simulink model "Opm"  (Simulink 8.4)
settings: Solver=ode45  StartTime=0.0  StopTime=10.0  RelTol=1e-3
undefined symbols (not defined in the file): Opm_stDiagnosisOverride, Opm_stEngControl, Opm_stIOErrorOverride, Opm_tiIOErrorDelay
libraries: simulink x1
settings Model: Creator=YAL9FE  LastModifiedBy=ric9fe
settings DebuggingCC: FcnCallInpInsideContextMsg=EnableAllAsWarning

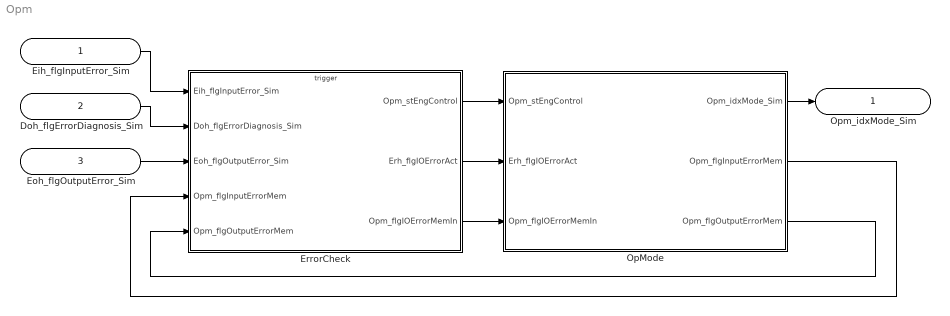
== system Opm ==
  Eih_flgInputError_Sim : Inport
  Doh_flgErrorDiagnosis_Sim : Inport  Port=2
  Eoh_flgOutputError_Sim : Inport  Port=3
  ErrorCheck : Subsystem  mask(Functions){}
      mask help: ErrorCheck
      mask Display:
      | image(imread('OperationMode.jpg'))
      | port_label('input',1,'Eih_flgInputError_Sim')
      | port_label('input',2,'Doh_flgErrorDiagnosis_Sim')
      | port_label('input',3,'Eoh_flgOutputError_Sim')
      | port_label('input',4,'Opm_flgInputErrorMem')
      | port_label('input',5,'Opm_flgOutputErrorMem')
      | port_label('output',1,'Opm_stEngControl')
      | port_label('output',2,'Erh_flgIOErrorAct')
      | port_label('output',3,'Opm_flgIOErrorMemIn')
  OpMode : Subsystem  mask(Functions){}
      mask help: OpMode
      mask Display:
      | image(imread('OperationMode.jpg'))
      | port_label('input',1,'Opm_stEngControl')
      | port_label('input',2,'Erh_flgIOErrorAct')
      | port_label('input',3,'Opm_flgIOErrorMemIn')
      | port_label('output',1,'Opm_idxMode_Sim')
      | port_label('output',2,'Opm_flgInputErrorMem')
      | port_label('output',3,'Opm_flgOutputErrorMem')
  Opm_idxMode_Sim : Outport
  wires:
  Eih_flgInputError_Sim/1 -> ErrorCheck/1(Eih_flgInputError_Sim)
  Doh_flgErrorDiagnosis_Sim/1 -> ErrorCheck/2(Doh_flgErrorDiagnosis_Sim)
  Eoh_flgOutputError_Sim/1 -> ErrorCheck/3(Eoh_flgOutputError_Sim)
  OpMode/1(Opm_idxMode_Sim) -> Opm_idxMode_Sim/1
  ErrorCheck/1(Opm_stEngControl) -> OpMode/1(Opm_stEngControl)
  ErrorCheck/2(Erh_flgIOErrorAct) -> OpMode/2(Erh_flgIOErrorAct)
  ErrorCheck/3(Opm_flgIOErrorMemIn) -> OpMode/3(Opm_flgIOErrorMemIn)
  OpMode/2(Opm_flgInputErrorMem) -> ErrorCheck/4(Opm_flgInputErrorMem)
  OpMode/3(Opm_flgOutputErrorMem) -> ErrorCheck/5(Opm_flgOutputErrorMem)

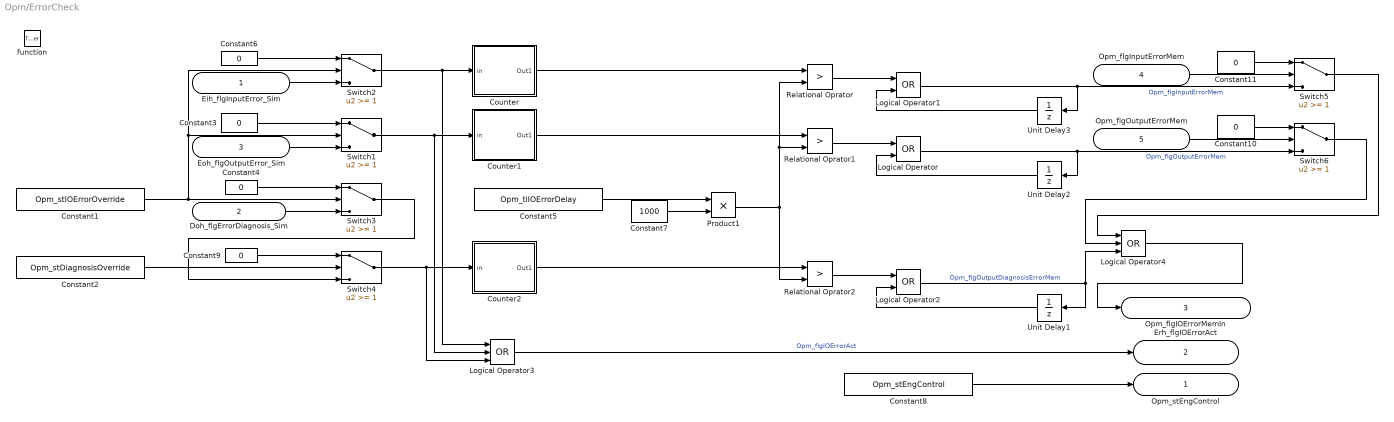
== system Opm/ErrorCheck ==
  Eih_flgInputError_Sim : Inport
  Doh_flgErrorDiagnosis_Sim : Inport  Port=2
  Eoh_flgOutputError_Sim : Inport  Port=3
  Opm_flgInputErrorMem : Inport  Port=4
  Opm_flgOutputErrorMem : Inport  Port=5
  function : TriggerPort  TriggerType=function-call
  Constant1 : Constant  Value=Opm_stIOErrorOverride
  Constant{3..4,6,9..11} (6 alike) : Constant  Value=0  OutDataTypeStr=boolean
  Constant2 : Constant  Value=Opm_stDiagnosisOverride
  Constant5 : Constant  Value=Opm_tiIOErrorDelay
  Constant7 : Constant  Value=1000  OutDataTypeStr=single
  Constant8 : Constant  Value=Opm_stEngControl
  Counter : Subsystem
      mask help: Counter
      mask Display: image(imread('Counter.jpg'))
  Counter1 : Subsystem
      mask help: Counter
      mask Display: image(imread('Counter.jpg'))
  Counter2 : Subsystem
      mask help: Counter
      mask Display: image(imread('Counter.jpg'))
  Logical Operator : Logic  Operator=OR  AllPortsSameDT=off  OutDataTypeStr=boolean
  Logical Operator1 : Logic  Operator=OR  AllPortsSameDT=off  OutDataTypeStr=boolean
  Logical Operator2 : Logic  Operator=OR  AllPortsSameDT=off  OutDataTypeStr=boolean
  Logical Operator3 : Logic  Operator=OR  Inputs=3  AllPortsSameDT=off  OutDataTypeStr=boolean
  Logical Operator4 : Logic  Operator=OR  Inputs=3  AllPortsSameDT=off  OutDataTypeStr=boolean
  Product1 : Product  OutDataTypeStr=Inherit: Same as first input
  Relational Oprator : RelationalOperator  Operator=>  OutDataTypeStr=boolean
  Relational Oprator1 : RelationalOperator  Operator=>  OutDataTypeStr=boolean
  Relational Oprator2 : RelationalOperator  Operator=>  OutDataTypeStr=boolean
  Switch{1..6} (6 alike) : Switch  Threshold=1
  Unit Delay1 : UnitDelay  SampleTime=-1
  Unit Delay2 : UnitDelay  SampleTime=-1
  Unit Delay3 : UnitDelay  SampleTime=-1
  Opm_stEngControl : Outport
  Erh_flgIOErrorAct : Outport  Port=2
  Opm_flgIOErrorMemIn : Outport  Port=3
  wires:
  Constant6/1 -> Switch2/1
  Constant1/1 -> Switch2/2, Switch1/2, Switch3/2
  Eih_flgInputError_Sim/1 -> Switch2/3
  Constant3/1 -> Switch1/1
  Constant4/1 -> Switch3/1
  Doh_flgErrorDiagnosis_Sim/1 -> Switch3/3
  Eoh_flgOutputError_Sim/1 -> Switch1/3
  Switch3/1 -> Switch4/3
  Constant9/1 -> Switch4/1
  Constant2/1 -> Switch4/2
  Switch2/1 -> Counter/1(in), Logical Operator3/1
  Switch1/1 -> Counter1/1(in), Logical Operator3/2
  Switch4/1 -> Counter2/1(in), Logical Operator3/3
  Constant5/1 -> Product1/1
  Constant7/1 -> Product1/2
  Counter/1(Out1) -> Relational Oprator/1
  Counter1/1(Out1) -> Relational Oprator1/1
  Product1/1 -> Relational Oprator/2, Relational Oprator1/2, Relational Oprator2/2
  Counter2/1(Out1) -> Relational Oprator2/1
  Relational Oprator/1 -> Logical Operator1/1
  Relational Oprator1/1 -> Logical Operator/1
  Relational Oprator2/1 -> Logical Operator2/1
  Logical Operator1/1 -> Unit Delay3/1, Switch5/3  "Opm_flgInputErrorMem"
  Unit Delay3/1 -> Logical Operator1/2
  Unit Delay2/1 -> Logical Operator/2
  Logical Operator/1 -> Unit Delay2/1, Switch6/3  "Opm_flgOutputErrorMem"
  Unit Delay1/1 -> Logical Operator2/2
  Logical Operator2/1 -> Unit Delay1/1, Logical Operator4/3  "Opm_flgOutputDiagnosisErrorMem"
  Logical Operator3/1 -> Erh_flgIOErrorAct/1  "Opm_flgIOErrorAct"
  Constant8/1 -> Opm_stEngControl/1
  Logical Operator4/1 -> Opm_flgIOErrorMemIn/1
  Constant11/1 -> Switch5/1
  Constant10/1 -> Switch6/1
  Opm_flgInputErrorMem/1 -> Switch5/2
  Opm_flgOutputErrorMem/1 -> Switch6/2
  Switch5/1 -> Logical Operator4/1
  Switch6/1 -> Logical Operator4/2

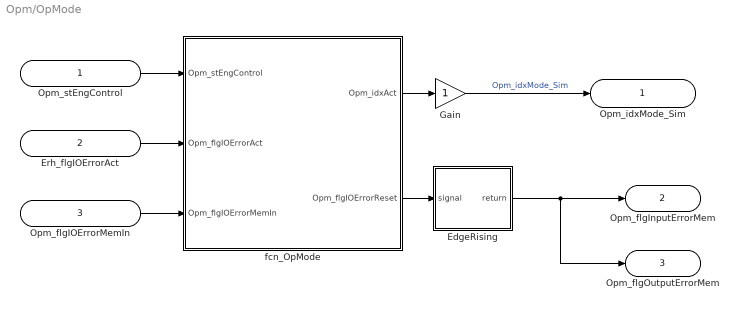
== system Opm/OpMode ==
  Opm_stEngControl : Inport
  Erh_flgIOErrorAct : Inport  Port=2
  Opm_flgIOErrorMemIn : Inport  Port=3
  EdgeRising : Subsystem
      mask help: EdgeRising
      mask Display: image(imread('EdgeRising.jpg'))
  Gain : Gain
  fcn_OpMode : MATLAB Function  TreatAsAtomicUnit=on
  Opm_idxMode_Sim : Outport
  Opm_flgInputErrorMem : Outport  Port=2
  Opm_flgOutputErrorMem : Outport  Port=3
  wires:
  Opm_stEngControl/1 -> fcn_OpMode/1(Opm_stEngControl)
  Erh_flgIOErrorAct/1 -> fcn_OpMode/2(Opm_flgIOErrorAct)
  Opm_flgIOErrorMemIn/1 -> fcn_OpMode/3(Opm_flgIOErrorMemIn)
  fcn_OpMode/1(Opm_idxAct) -> Gain/1
  fcn_OpMode/2(Opm_flgIOErrorReset) -> EdgeRising/1(signal)
  Gain/1 -> Opm_idxMode_Sim/1  "Opm_idxMode_Sim"
  EdgeRising/1(return) -> Opm_flgInputErrorMem/1, Opm_flgOutputErrorMem/1

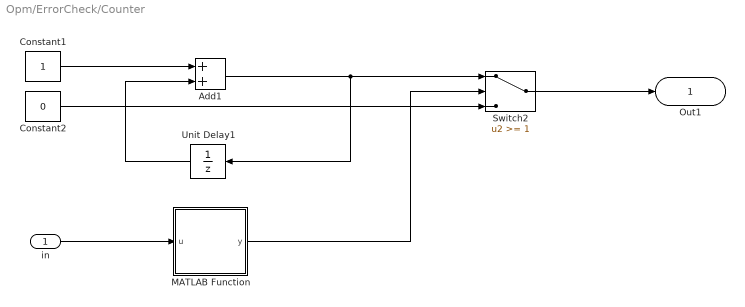
== system Opm/ErrorCheck/Counter ==
  in : Inport
  Add1 : Sum
  Constant1 : Constant  OutDataTypeStr=single
  Constant2 : Constant  Value=0  OutDataTypeStr=single
  MATLAB Function : MATLAB Function  TreatAsAtomicUnit=on
  Switch2 : Switch  Threshold=1
  Unit Delay1 : UnitDelay  SampleTime=-1
  Out1 : Outport
  wires:
  in/1 -> MATLAB Function/1(u)
  MATLAB Function/1(y) -> Switch2/2
  Add1/1 -> Unit Delay1/1, Switch2/1
  Constant2/1 -> Switch2/3
  Switch2/1 -> Out1/1
  Unit Delay1/1 -> Add1/2
  Constant1/1 -> Add1/1

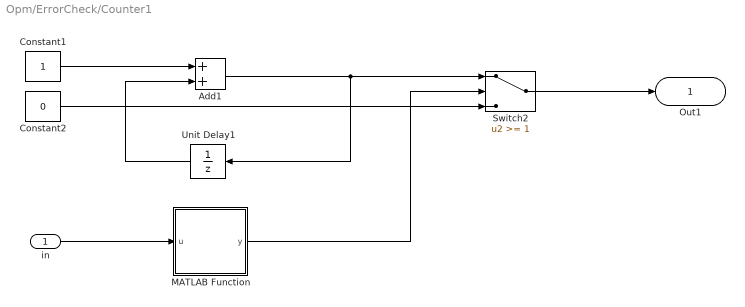
== system Opm/ErrorCheck/Counter1 ==
  in : Inport
  Add1 : Sum
  Constant1 : Constant  OutDataTypeStr=single
  Constant2 : Constant  Value=0  OutDataTypeStr=single
  MATLAB Function : MATLAB Function  TreatAsAtomicUnit=on
  Switch2 : Switch  Threshold=1
  Unit Delay1 : UnitDelay  SampleTime=-1
  Out1 : Outport
  wires:
  Constant1/1 -> Add1/1
  Unit Delay1/1 -> Add1/2
  Switch2/1 -> Out1/1
  Constant2/1 -> Switch2/3
  Add1/1 -> Switch2/1, Unit Delay1/1
  MATLAB Function/1(y) -> Switch2/2
  in/1 -> MATLAB Function/1(u)

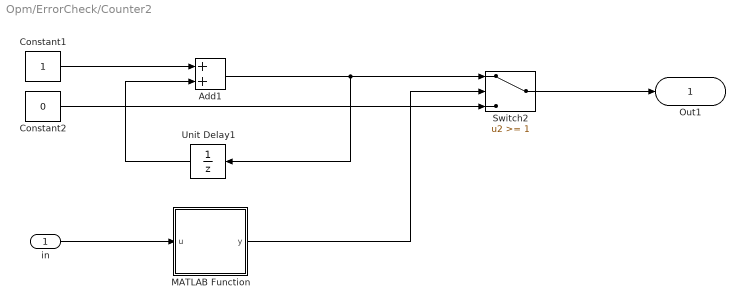
== system Opm/ErrorCheck/Counter2 ==
  in : Inport
  Add1 : Sum
  Constant1 : Constant  OutDataTypeStr=single
  Constant2 : Constant  Value=0  OutDataTypeStr=single
  MATLAB Function : MATLAB Function  TreatAsAtomicUnit=on
  Switch2 : Switch  Threshold=1
  Unit Delay1 : UnitDelay  SampleTime=-1
  Out1 : Outport
  wires:
  in/1 -> MATLAB Function/1(u)
  MATLAB Function/1(y) -> Switch2/2
  Add1/1 -> Unit Delay1/1, Switch2/1
  Constant2/1 -> Switch2/3
  Switch2/1 -> Out1/1
  Unit Delay1/1 -> Add1/2
  Constant1/1 -> Add1/1

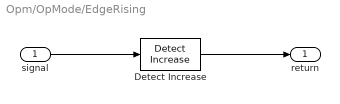
== system Opm/OpMode/EdgeRising ==
  signal : Inport
  Detect Increase : simulink/Logic and Bit Operations/Detect Increase  vinit=0.0  InputProcessing=Inherited  OutDataTypeStr=boolean
  return : Outport
  wires:
  signal/1 -> Detect Increase/1
  Detect Increase/1 -> return/1

== matlab function OpMode/fcn_OpMode ==
  data: Opm_stEngControl input double; Opm_flgIOErrorAct input double; Opm_idxAct output double; Opm_flgIOErrorMemIn input double; Opm_flgIOErrorReset output double
function [Opm_idxAct,Opm_flgIOErrorReset]= fcn(Opm_stEngControl,Opm_flgIOErrorAct,Opm_flgIOErrorMemIn)
% fcn_OpMode

sm = single(0);
Opm_idxAct = single(0);
Opm_flgIOErrorReset = false;

if(sm==0)                                            % Off_state
        if(Opm_stEngControl)
            Opm_idxAct = single(1);
            sm = single(2);
        end
        if(Opm_flgIOErrorMemIn)
            Opm_idxAct = single(2);
            sm = single(1);
        end
        Opm_flgIOErrorReset = false;
end
if(sm==1)                                            % IOError_state
        if((~Opm_stEngControl)&&(~Opm_flgIOErrorAct))
            Opm_flgIOErrorReset = true;
            Opm_idxAct = single(0);
            sm = single(0);
        end
end
if(sm==2)                                            % Normal_state
        if(~Opm_stEngControl)
            Opm_idxAct = single(0);
            sm = single(0);
        end
        if(Opm_flgIOErrorMemIn)
            Opm_idxAct = single(2);
            sm = single(1);
        end
        Opm_flgIOErrorReset = false;
end

== matlab function ErrorCheck/Counter/MATLAB Function ==
  data: u input double; y output double
function y = fcn(u)
% initValue Test
if(u<=0)
    y = 0;
else
    y = 1;
end

== matlab function ErrorCheck/Counter1/MATLAB Function ==
  data: u input double; y output double
function y = fcn(u)
% initValue Test
if(u<=0)
    y = 0;
else
    y = 1;
end

== matlab function ErrorCheck/Counter2/MATLAB Function ==
  data: u input double; y output double
function y = fcn(u)
% initValue Test
if(u<=0)
    y = 0;
else
    y = 1;
end
